simulink library "CrossFaderLib"  (R2022b)
settings: Solver=VariableStepAuto  StartTime=0.0  StopTime=10.0  RelTol=1e-3
libraries: AudioStats x1, HandyTextFile x1
settings Model: Creator=jb1046154  LastModifiedBy=sa1045272
settings SolverCC: AlgebraicLoopSolver=TrustRegion
settings DebuggingCC: UnconnectedInputMsg=warning  UnconnectedOutputMsg=warning  UnconnectedLineMsg=warning  SFMachineParentedDataDiag=warning
settings ModelReferenceCC: EnableRefExpFcnMdlSchedulingChecks=on

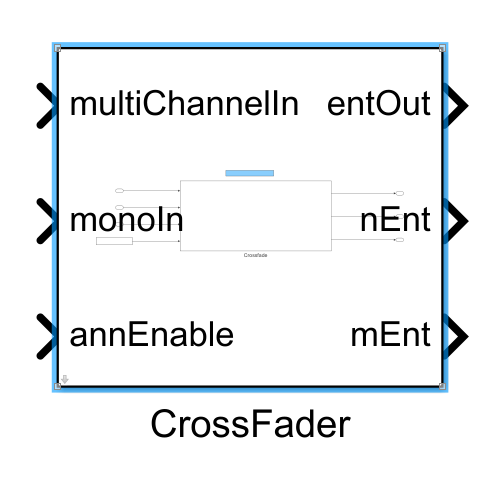
[thumbnail: Simulink's stored preview of the top-level diagram]
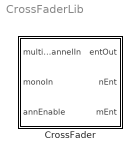
== system CrossFaderLib ==
  CrossFader : Subsystem  mask(Crossfader){Config=[]}
      mask prompts: Config "CrossFaderConfig"
      mask help:
      | This mask allows the setting of parameters for the Crossfader model.
      | Model parameters are set by a class instance in the base workspace.
      |
      | See 'Help' for details.
      mask init:
      | blkh=gcbh;
      | Config=BTConfig.Assert(blkh,Config);
      | 
      | Config.Validate();
      | Config.DoMaskInit(blkh);
      settings: LibrarySourceBlock=PreAmpLib/PreAmp/Subsystem
      mask Help:
      | Defining model parameters:
      | The model parameters are set by the conents of an instance of CrossfaderClass.m.
      | 
      | To set model parameters:
      | 1-Create an instance of CrossfaderClass.m in the base workspace.
      | 2-In the model mask, set the 'Class instance' parameter to the name of the class instance in the base workspace.

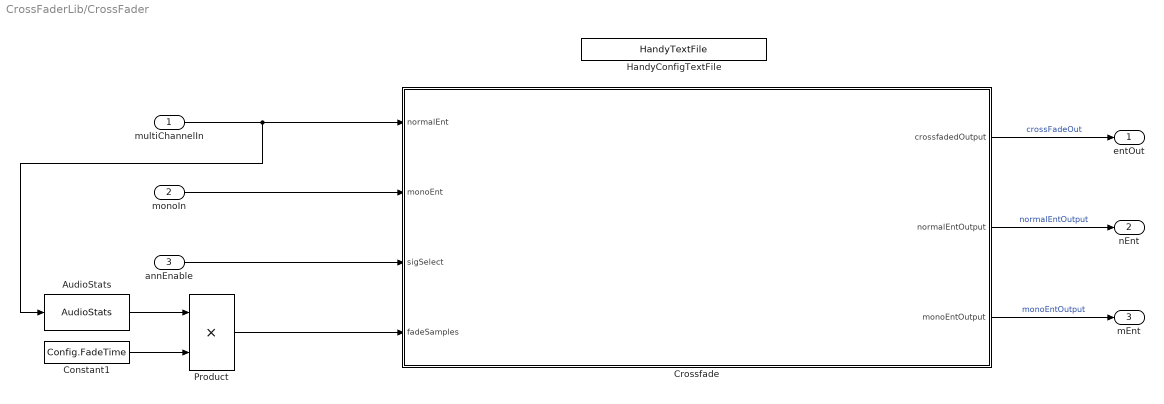
== system CrossFaderLib/CrossFader ==
  multiChannelIn : Inport
  monoIn : Inport  Port=2
  annEnable : Inport  Port=3
  AudioStats : AudioStats/AudioStats  DoSampleRate=on  TypeSampleRate=Inherit: auto  DoCallRate=off  TypeCallRate=Inherit: auto  DoFrameSize=off  TypeFrameSize=Inherit: auto  DoChannelCount=off  TypeChannelCount=Inherit: auto  DoTaskRateFactor=off  TypeTaskRateFactor=Inherit: auto  MacroNameRoot=AUDIO  MacroNameRootEval='AUDIO'  IsMacroNameEval=off  MacroSampleRate=off  MacroCallRate=off  MacroFrameSize=off  MacroChannelCount=off  MacroTaskRateFactor=off  MacroTaskId=off  ValidateSampleRate=off  ValueSampleRate=[]  ValidateCallRate=off  ValueCallRate=[]  ValidateFrameSize=off  ValueFrameSize=[]  ValidateChannelCount=off  ValueChannelCount=[]  ValidateTaskRateFactor=off  ValueTaskRateFactor=[]
      settings: SourceProductName=Bose Talaria
  Constant1 : Constant  Value=Config.FadeTime
  "Crossfade " : MATLAB Function  TreatAsAtomicUnit=on
  HandyConfigTextFile : HandyTextFile/HandyTextFile  TemplateSource=Config  FileSuffix=File  OpenDialogOnLoad=off  UseThisBlockName=off  AddGrandParentNamePrefix=off  TheDefaultText=% $(FILENAME) $(PREFIX) $(SUFFIX)  ShowInLibBrowser=on
      settings: SourceProductName=Bose Talaria
  Product : Product
  entOut : Outport
  nEnt : Outport  Port=2
  mEnt : Outport  Port=3
  wires:
  "Crossfade "/1(crossfadedOutput) -> entOut/1  "crossFadeOut"
  monoIn/1 -> "Crossfade "/2(monoEnt)
  multiChannelIn/1 -> AudioStats/1, "Crossfade "/1(normalEnt)
  Product/1 -> "Crossfade "/4(fadeSamples)
  annEnable/1 -> "Crossfade "/3(sigSelect)
  "Crossfade "/2(normalEntOutput) -> nEnt/1  "normalEntOutput"
  "Crossfade "/3(monoEntOutput) -> mEnt/1  "monoEntOutput"
  Constant1/1 -> Product/2
  AudioStats/1 -> Product/1

== matlab function CrossFaderLib/CrossFader/Crossfade  ==
  data: normalEnt input; crossfadedOutput output; monoEnt input; sigSelect input; fadeSamples input; normalEntOutput output; monoEntOutput output
function [crossfadedOutput, normalEntOutput, monoEntOutput] = crossfade(normalEnt,monoEnt,sigSelect,fadeSamples)
% fadetime in ms
% sigSelect = 0 passes normalEnt, sigSelect = 1 passes monoEnt

persistent currentFadeInd;
persistent currentSig;

% first run init
if (isempty(currentFadeInd))
    currentFadeInd = 0;
    currentSig = uint32(0);
end

% Selection changed
startFade = 0;
if (currentSig ~= sigSelect)
%    currentSig = sigSelect;
    currentSig = uint32(sigSelect);
    currentFadeInd = 0;
    startFade = 1;
end

crossfadedOutput = single(zeros(size(normalEnt)));
normalEntOutput = single(zeros(size(normalEnt)));
monoEntOutput = single(zeros(size(normalEnt)));

% Process the audio
if ((currentFadeInd ~= 0)||(startFade))
    % Apply the cross fade gains, either because we're mid-ramp or we're
    % starting over
    for (samp = 1:size(normalEnt, 1))
        currentFadeInd = currentFadeInd + 1;
        % lookup gains for this sample
        if (currentFadeInd > fadeSamples)
            % we hit the end of the ramp, but we're still working
            % a frame that was ramping
            if (currentSig)
                normalEntGain = 0;
                monoEntGain = 1;
            else
                normalEntGain = 1;
                monoEntGain = 0;
            end
        else
            % actively ramping
            if (currentSig)
%                 sig1Gain = fadeDownGain(currentFadeInd);
                normalEntGain = 1-(currentFadeInd/fadeSamples);
%                 sig2Gain = fadeUpGain(currentFadeInd);
                monoEntGain = (currentFadeInd/fadeSamples);
            else
%                 sig1Gain = fadeUpGain(currentFadeInd);
                normalEntGain = (currentFadeInd/fadeSamples);
%                 sig2Gain = fadeDownGain(currentFadeInd);
                monoEntGain = 1-(currentFadeInd/fadeSamples);
            end
        end
        % apply gains
        normalEntOutput(samp,:) = (normalEnt(samp,:)*normalEntGain);
        monoEntOutput(samp,:) = (monoEnt(samp,:)*monoEntGain);
        crossfadedOutput(samp,:) = single(normalEnt(samp,:)*normalEntGain + monoEnt(samp,:)*monoEntGain);
    end
    % reset fade if finished
    if (currentFadeInd > fadeSamples)
        currentFadeInd = 0;
    end
else
    % Just pass selected signal
    if (currentSig)
        crossfadedOutput = single(monoEnt(1:size(normalEnt,1),1:size(normalEnt,2)));
    else
        crossfadedOutput = single(normalEnt);
    end
end
